simulink model "dc_ac_converter_simulation"  (R2023a)
settings: Solver=VariableStepAuto  StartTime=0.0  StopTime=sim_time  RelTol=1e-3
values from neighbouring files (symbols this model uses):
  gridfreq_rad = 2*pi*gridfreq    (= 314.159265359)    [dc_ac_converter_script.m]
  modulation = 0.8    [dc_ac_converter_script.m]
  modulation_angle = 0.123    [dc_ac_converter_script.m]
  Rd = 0.1    [dc_ac_converter_script.m]
  solver_sample_time = (1/Carrier_freq_modulation)/100    (= 6.06060606061e-06)    [dc_ac_converter_script.m]
  Vd = 3010    [dc_ac_converter_script.m]
libraries: fl_lib x22, nesl_utility x16, ee_lib x7, eeGeneralControl x6, spsTriangleGeneratorLib x1
settings Model: Creator=citcea  LastModifiedBy=citcea

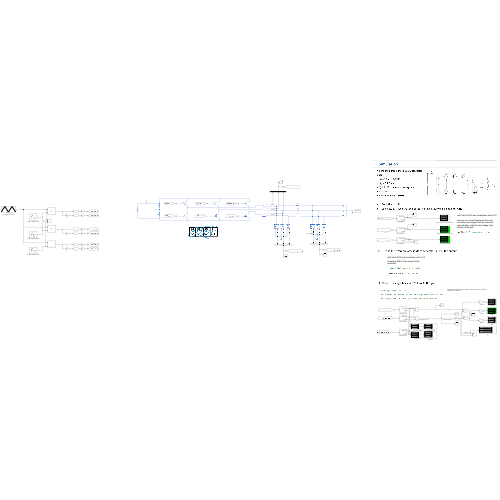
[thumbnail: Simulink's stored preview of the top-level diagram]
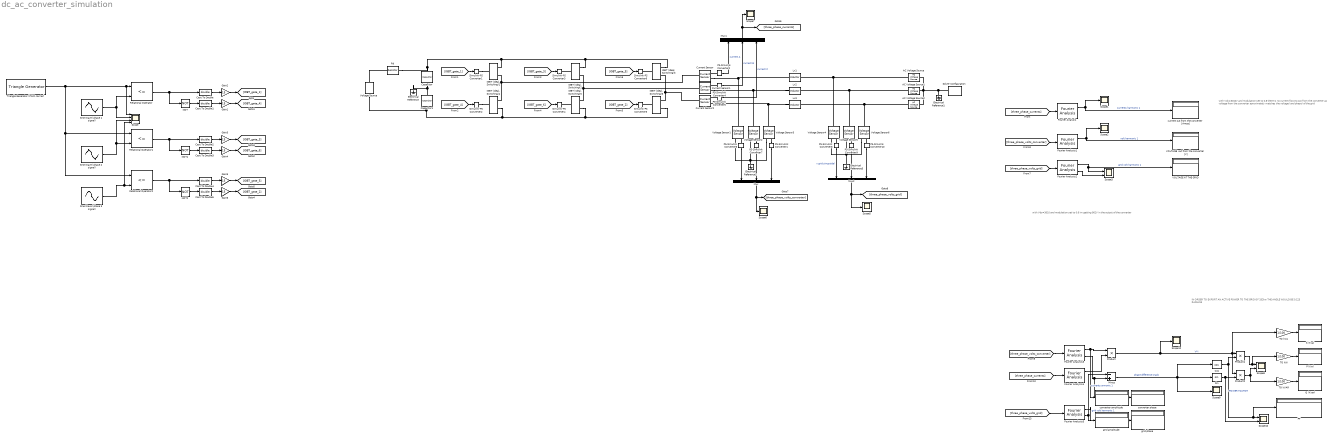
== system dc_ac_converter_simulation ==
  note: IN ORDER TO EXPORT AN ACTIVE POWER TO THE GRID OF 202kw THE ANGLE WOULD BE 0.123 RADIANS
  note: with Vdc=3010 and modulation set to 0.6
      |
      | im getting 902V in the output of the converter
  note: with Vdc=3010V and modulation set to 0.8
      |
      | there is no current flowing out from the converter as voltage from the converter aproximately matches the voltage (and phase) of the grid
  AC Voltage Source : fl_lib/Electrical/Electrical Sources/AC Voltage Source  amp=Vspeak_phase_to_ground V  shift=0 deg  frequency=gridfreq Hz  omega=0 rad/s
  AC Voltage Source1 : fl_lib/Electrical/Electrical Sources/AC Voltage Source  amp=Vspeak_phase_to_ground V  shift=120 deg  frequency=gridfreq Hz  omega=0 rad/s
  AC Voltage Source2 : fl_lib/Electrical/Electrical Sources/AC Voltage Source  amp=Vspeak_phase_to_ground V  shift=120*2 deg  frequency=gridfreq Hz  omega=0 rad/s
  Capacitor : fl_lib/Electrical/Electrical Elements/Capacitor  c=C F  r=1e-6 Ohm  g=0 1/Ohm  i_specify=off  i_priority=None  i=0 A  i_nominal_specify=off  i_nominal_unit=A  i_nominal_value=1  v_specify=off  v_priority=None  v=0 V  v_nominal_specify=off  v_nominal_unit=V  v_nominal_value=1  vc_specify=on  vc_priority=High  vc=Vd/2 V  vc_nominal_specify=off  vc_nominal_unit=V  vc_nominal_value=1
  Capacitor1 : fl_lib/Electrical/Electrical Elements/Capacitor  c=C F  r=1e-6 Ohm  g=0 1/Ohm  i_specify=off  i_priority=None  i=0 A  i_nominal_specify=off  i_nominal_unit=A  i_nominal_value=1  v_specify=off  v_priority=None  v=0 V  v_nominal_specify=off  v_nominal_unit=V  v_nominal_value=1  vc_specify=on  vc_priority=High  vc=Vd/2 V  vc_nominal_specify=off  vc_nominal_unit=V  vc_nominal_value=1
  Cast To Double{,1..5} (6 alike) : DataTypeConversion  OutDataTypeStr=double  SaturateOnIntegerOverflow=off  RndMeth=Floor
  Cos : Trigonometry  Operator=cos
  Current Sensor : fl_lib/Electrical/Electrical Sensors/Current Sensor
  Current Sensor1 : fl_lib/Electrical/Electrical Sensors/Current Sensor
  Current Sensor2 : fl_lib/Electrical/Electrical Sensors/Current Sensor
  Electrical Reference{,1..3} (4 alike) : fl_lib/Electrical/Electrical Elements/Electrical Reference
  Fourier Analysis{,1..5} (6 alike) : eeGeneralControl/Fourier Analysis  f=gridfreq  n=[1]  M0=0  Ph0=0  BufferSize=8192  Ts=solver_sample_time
      settings: LibrarySourceBlock=ee_sl_lib/General Control/Fourier Analysis
  Gain{1..6} (6 alike) : Gain  Gain=15
  IGBT (Ideal, Switching){1..6} (6 alike) : ee_lib/Semiconductors & Converters/IGBT (Ideal, Switching)  port_option=ee.enum.controlport.ps  Vf=0.8 V  Ron=0.001 Ohm  Goff=1e-5 1/Ohm  Vth=6 V  diode_param=ee.enum.converters.protectiondiode.nodynamics  diode_Vf=0.8 V  diode_Ron=0.001 Ohm  diode_Goff=1e-5 1/Ohm  diode_C=50e-9 F  diode_iRM=-235 A  diode_iF=300 A  diode_idot=-50 A/us  diode_trr_param=ee.enum.converters.diodeReverseParam.trr_factor  diode_trr_factor=3  diode_trr=15 us  diode_Qrr=1500 s*uA  ice_specify=off  ice_priority=None  ice=0 A  ice_nominal_specify=off  ice_nominal_unit=A  ice_nominal_value=1  vce_specify=off  vce_priority=None  vce=0 V  vce_nominal_specify=off  vce_nominal_unit=V  vce_nominal_value=1  vge_specify=off  vge_priority=None  vge=0 V  vge_nominal_specify=off  vge_nominal_unit=V  vge_nominal_value=1  thermal_loss_option=ee.enum.converters.thermalLossOption.constantvalues  Von_data=[0, .1, .6, .8, 1, 1.3, 1.6, 2, 2.4; 0, .1, .7, 1, 1.2, 1.5, 1.9, 2.4, 2.8] V  Tj=[298.15, 398.15] K  Iout_data=[0, .1, 1, 5, 10, 20, 40, 70, 100] A  Eon_data=[0, .0024, .024, .12, .2, .48, 1.04, 2.16, 3.24; 0, .003, .03, .15, .25, .6, 1.3, 2.7, 4.05] * 1e-3 J  Eoff_data=[0, .0007, .0066, .033, .066, .17, .33, .83, 1.5; 0, .001, .01, .05, .1, .25, .5, 1.2, 2.2] * 1e-3 J  Tj_loss=[298.15, 398.15] K  Iout_data_loss=[0, .1, 1, 5, 10, 20, 40, 70, 100] A  Eon_scalar=22.86e-3 J  Eoff_scalar=17.14e-3 J  Voff=300 V  Iout_scalar=600 A  diodeModelType=ee.enum.converters.diodeModelType.pwl  diodeTableType=ee.enum.diode.tableType.IfMat  diode_IfMat=[.07, .12, .19, 1.75, 4.24, 7.32, 11.2; .16, .3, .72, 2.14, 4.02, 6.35, 9.12] A  diode_VfMat=[.9, 1.15, 1.25, 1.5, 1.75, 2.17, 2.6, 2.85; .58, .68, .75, 1.1, 1.38, 1.77, 2.27, 2.7] V  diode_TjVec=[25, 125] degC  diode_VfVec=[.5, .7, .9, 1.3, 1.7, 2.1, 2.5] V  diode_IfVec=[.1, .2, .5, 1, 2, 4, 7, 10] A  diode_Vr=-600 V  diode_Ls=150 nH  diode_Erec=0.03 J  diode_rec_loss_model=ee.enum.diode.reverseRecoveryModel.fixed  diode_ErecVal=0 J  diode_ErecMat=zeros(2, 3) J  diode_TjrecVec=[298.15, 398.15] K  diode_IfrecVec=[.1, 1, 10] A  diode_VrecVal=10 V  diode_tFilter=1 / 1000 / 100 s  thermal_network_parameterization=ee.enum.thermalNetworkTopology.external  Rth=[.08, .5] K/W  Rth_Cauer=[.08, .1, .5] K/W  Rth_Foster=[.08, .14, .22, .16] K/W  thermal_mass_parameterization=ee.enum.thermalNetwork.timeconstant  thermal_mass=[.01, .5] J/K  thermal_mass_Cauer=[.01, .1, .5] J/K  thermal_mass_Foster=[.001, .005, .05, .5] J/K  thermal_time_constant=[.001, .2] s  thermal_time_constant_Cauer=[.001, .1, .2] s  thermal_time_constant_Foster=[7e-05, .0007, .01, .08] s  thermal_mass_initial_temperatures=[25, 25] degC  thermal_mass_initial_temperatures_Cauer=[25, 25, 25] degC  junction_thermal_mass=0.01 J/K  Tvec_initial_Foster=[25, 25, 25, 25] degC  no_thermal_network=0  junction_temperature_specify=off  junction_temperature_priority=None  junction_temperature=25 degC  junction_temperature_nominal_specify=off  junction_temperature_nominal_unit=degC  junction_temperature_nominal_value=1  Qj_specify=off  Qj_priority=None  Qj=0 W  Qj_nominal_specify=off  Qj_nominal_unit=W  Qj_nominal_value=1
  Lx1 : fl_lib/Electrical/Electrical Elements/Inductor  l=Ls H  r=RLs Ohm  g=1e-9 1/Ohm  i_specify=off  i_priority=None  i=0 A  i_nominal_specify=off  i_nominal_unit=A  i_nominal_value=1  v_specify=off  v_priority=None  v=0 V  v_nominal_specify=off  v_nominal_unit=V  v_nominal_value=1  i_L_specify=off  i_L_priority=High  i_L=0 A  i_L_nominal_specify=off  i_L_nominal_unit=A  i_L_nominal_value=1
  Lx2 : fl_lib/Electrical/Electrical Elements/Inductor  l=Ls H  r=RLs Ohm  g=1e-9 1/Ohm  i_specify=off  i_priority=None  i=0 A  i_nominal_specify=off  i_nominal_unit=A  i_nominal_value=1  v_specify=off  v_priority=None  v=0 V  v_nominal_specify=off  v_nominal_unit=V  v_nominal_value=1  i_L_specify=off  i_L_priority=High  i_L=0 A  i_L_nominal_specify=off  i_L_nominal_unit=A  i_L_nominal_value=1
  Lx3 : fl_lib/Electrical/Electrical Elements/Inductor  l=Ls H  r=RLs Ohm  g=1e-9 1/Ohm  i_specify=off  i_priority=None  i=0 A  i_nominal_specify=off  i_nominal_unit=A  i_nominal_value=1  v_specify=off  v_priority=None  v=0 V  v_nominal_specify=off  v_nominal_unit=V  v_nominal_value=1  i_L_specify=off  i_L_priority=High  i_L=0 A  i_L_nominal_specify=off  i_L_nominal_unit=A  i_L_nominal_value=1
  Minus : Sum  Inputs=-+
  Mux : Mux  Inputs=3
  Mux1 : Mux  Inputs=3
  Mux2 : Mux  Inputs=3
  NOT : Logic  Operator=NOT  IconShape=distinctive  AllPortsSameDT=off  OutDataTypeStr=boolean
  NOT1 : Logic  Operator=NOT  IconShape=distinctive  AllPortsSameDT=off  OutDataTypeStr=boolean
  NOT2 : Logic  Operator=NOT  IconShape=distinctive  AllPortsSameDT=off  OutDataTypeStr=boolean
  P (Kw) : Display
  PF : Display
  PS-Simulink Converter{1..2,4..10} (9 alike) : nesl_utility/PS-Simulink Converter  PhysicalDomain=network_engine_domain  SubClassName=ps_output  LeftPortType=input  RightPortType=output  PseudoPeriodic=off  Frequencies=[]  VectorFormat=inherit  Unit=inherit  AffineConversion=off
  Product : Product
  Product1 : Product
  Product2 : Product
  Q (Kvar) : Display
  Rd : fl_lib/Electrical/Electrical Elements/Resistor  R=Rd Ohm  i_specify=off  i_priority=None  i=0 A  i_nominal_specify=off  i_nominal_unit=A  i_nominal_value=1  v_specify=off  v_priority=None  v=0 V  v_nominal_specify=off  v_nominal_unit=V  v_nominal_value=1
  Relational Operator : RelationalOperator  Operator=<=  OutDataTypeStr=boolean  RndMeth=Simplest  InputSameDT=off
  Relational Operator1 : RelationalOperator  Operator=<=  OutDataTypeStr=boolean  RndMeth=Simplest  InputSameDT=off
  Relational Operator2 : RelationalOperator  Operator=<=  OutDataTypeStr=boolean  RndMeth=Simplest  InputSameDT=off
  S (Kva) : Display
  Scope : Scope  NumInputPorts=4
  Scope{1..2,5..7,9,12} (7 alike) : Scope
  Scope10 : Scope  NumInputPorts=2
  Scope3 : Scope  NumInputPorts=2
  Scope8 : Scope  NumInputPorts=2
  Simulink-PS Converter{1..6} (6 alike) : nesl_utility/Simulink-PS Converter  PhysicalDomain=network_engine_domain  SubClassName=ps_input  LeftPortType=input  RightPortType=output  PseudoPeriodic=off  Frequencies=[]  NoiseDistribution=none  NoiseParameters=[]  Unit=1  AffineConversion=off  FilteringAndDerivatives=provide  SimscapeFilterOrder=1  InputFilterTimeConstant=0.001  UdotUserProvided=0
  Sin : Trigonometry
  Sine Wave (phase 1 signal) : Sin  Amplitude=modulation  Frequency=gridfreq_rad  Phase=modulation_angle  SampleTime=0
  Sine Wave (phase 2 signal) : Sin  Amplitude=modulation  Frequency=gridfreq_rad  Phase=(120*pi/180)+modulation_angle  SampleTime=0
  Sine Wave (phase 3 signal) : Sin  Amplitude=modulation  Frequency=gridfreq_rad  Phase=(240*pi/180)+modulation_angle  SampleTime=0
  Solver Configuration : nesl_utility/Solver Configuration  PhysicalDomain=network_engine_domain  SubClassName=solver  LeftPortType=input  RightPortType=generic  Tones=[]  Harmonics=[]  SimulateNoise=off  Profile=off  UseLocalSampling=off  EnableSwitchedLinearOptims=on  FrequencyDomain=off  UseCCode=off  RelTol=0.001  AbsTol=0.001  MinStep=1e-09  ToWorkspace=off  RevertToSquareIcSolve=off  NumHomotopyIterations=100  PhasorMode=off  PhasorModeNumHarmonics=1  ConsistencySolver=NEWTON_XTOL_AFTER_FTOL  IndexReductionMethod=DerivativeReplacement  DoDC=off  ResidualTolerance=1e-09  ConsistencyTolSource=GLOBAL  ConsistencyAbsTol=0.001  ConsistencyRelTol=0.001  ConsistencyTolFactor=0.001  UseLocalSolver=on  LocalSolverChoice=NE_BACKWARD_EULER_ADVANCER  ResolveIndetEquations=on  FunctionEvalNumThread=1  LocalSolverSampleTime=solver_sample_time  DoFixedCost=on  MaxNonlinIter=3  MaxModeIter=2  ComputeImpulses=off  ImpulseIterations=2  LinearAlgebra=auto  LinearAlgebraNumThread=0  EquationFormulation=NE_TIME_EF  DelaysMemoryBudget=1024  AutomaticFiltering=on  FilteringTimeConstant=0.001  PartitionStorageMethod=AS_NEEDED  PartitionMemoryBudget=1024  PartitionMethod=ROBUST
  TO kVA : Gain  Gain=1/100
  TO kVAR : Gain  Gain=1/100
  TO kW : Gain  Gain=1/100
  Triangle Generator (PWM carrier) : spsTriangleGeneratorLib/Triangle Generator  Freq=Carrier_freq_modulation  Phase=0  Ts=0
  VOLTAGE  out from the converter [V] : Display
  VOLTAGE AT THE GRID : Display
  Voltage Sensor{1..6} (6 alike) : fl_lib/Electrical/Electrical Sensors/Voltage Sensor
  Voltage Source : ee_lib/Sources/Voltage Source  dc_voltage=Vd V  ac_voltage=0 V  ac_shift=0 rad  ac_frequency=60 Hz  noise_mode=ee.enum.sources.noise.Disabled  PSD=0 V^2/Hz  sample_time=1e-3 s  repeatability=ee.enum.sources.repeatability.NotRepeatable  user_seed=0  auto_seed=3890346746  i_specify=off  i_priority=None  i=0 A  i_nominal_specify=off  i_nominal_unit=A  i_nominal_value=1  v_specify=off  v_priority=None  v=0 V  v_nominal_specify=off  v_nominal_unit=V  v_nominal_value=1
  converter amplitude : Display
  converter phase : Display
  current out from the converter [Amps] : Display
  grid amplitude : Display
  grid phase : Display
  wires:
  [IGBT_gate_1] -> Simulink-PS Converter1/1
  [IGBT_gate_4] -> Simulink-PS Converter2/1
  [IGBT_gate_3] -> Simulink-PS Converter3/1
  [IGBT_gate_6] -> Simulink-PS Converter4/1
  [IGBT_gate_2] -> Simulink-PS Converter5/1
  [IGBT_gate_5] -> Simulink-PS Converter6/1
  Sine Wave (phase 1 signal)/1 -> Scope/2, Relational Operator/2
  Relational Operator/1 -> Cast To Double/1, NOT/1
  Relational Operator1/1 -> Cast To Double2/1, NOT1/1
  Sine Wave (phase 2 signal)/1 -> Scope/3, Relational Operator1/2
  Relational Operator2/1 -> Cast To Double4/1, NOT2/1
  Sine Wave (phase 3 signal)/1 -> Scope/4, Relational Operator2/2
  Triangle Generator (PWM carrier)/1 -> Relational Operator2/1, Relational Operator1/1, Scope/1, Relational Operator/1
  NOT/1 -> Cast To Double1/1
  NOT1/1 -> Cast To Double3/1
  NOT2/1 -> Cast To Double5/1
  Cast To Double/1 -> Gain2/1
  Cast To Double1/1 -> Gain1/1
  Cast To Double2/1 -> Gain3/1
  Cast To Double3/1 -> Gain4/1
  Cast To Double4/1 -> Gain5/1
  Cast To Double5/1 -> Gain6/1
  Gain2/1 -> [IGBT_gate_1]
  Gain1/1 -> [IGBT_gate_4]
  Gain3/1 -> [IGBT_gate_3]
  Gain4/1 -> [IGBT_gate_6]
  Gain5/1 -> [IGBT_gate_5]
  Gain6/1 -> [IGBT_gate_2]
  PS-Simulink Converter5/1 -> Mux1/3  "current C"
  PS-Simulink Converter6/1 -> Mux/1
  PS-Simulink Converter7/1 -> Mux/2
  PS-Simulink Converter1/1 -> Mux/3
  PS-Simulink Converter8/1 -> Mux2/1  "v grid sinusoidal"
  PS-Simulink Converter9/1 -> Mux2/2
  PS-Simulink Converter2/1 -> Mux1/1  "current A"
  Mux1/1 -> Scope7/1, [three_phase_currents]
  Mux/1 -> Scope6/1, [three_phase_volts_converter]
  PS-Simulink Converter4/1 -> Mux1/2  "current B"
  PS-Simulink Converter10/1 -> Mux2/3
  Mux2/1 -> Scope5/1, [three_phase_volts_grid]
  [three_phase_currents] -> Fourier Analysis/1
  Fourier Analysis/1 -> Scope1/1, current out from the converter [Amps]/1  "currents harmonic 1"
  [three_phase_volts_converter] -> Fourier Analysis1/1
  [three_phase_volts_grid] -> Fourier Analysis2/1
  Fourier Analysis1/1 -> Scope2/1, VOLTAGE  out from the converter [V]/1  "volt harmonic 1"
  Fourier Analysis2/1 -> Scope3/1, VOLTAGE AT THE GRID/1  "grid volt harmonic 1"
  [three_phase_volts_converter] -> Fourier Analysis3/1
  [three_phase_currents] -> Fourier Analysis4/1
  Fourier Analysis4/1 -> Product/2
  Fourier Analysis3/1 -> converter amplitude/1, Product/1  "currents armonic 1"
  Product/1 -> Scope12/1, TO kVA/1, Product2/1, Product1/1  "V*I"
  Cos/1 -> PF/1, Scope10/1, Product1/2  "POWER FACTOR"
  Sin/1 -> Scope10/2, Product2/2
  Product1/1 -> Scope8/1, TO kW/1
  Product2/1 -> Scope8/2, TO kVAR/1
  Minus/1 -> Scope9/1, Sin/1, Cos/1  "phase difference [rad]"
  Fourier Analysis2/2 -> Scope3/2
  [three_phase_volts_grid] -> Fourier Analysis5/1
  Fourier Analysis3/2 -> converter phase/1, Minus/2
  Fourier Analysis5/2 -> grid phase/1, Minus/1
  Fourier Analysis5/1 -> grid amplitude/1  "grid volt harmonic 1"
  TO kW/1 -> P (Kw)/1
  TO kVA/1 -> S (Kva)/1
  TO kVAR/1 -> Q (Kvar)/1
  connections:
  Capacitor/RConn1 -- Electrical Reference/LConn1 -- Capacitor1/LConn1
  Rd/LConn1 -- "IGBT (Ideal, Switching)3"/RConn1 -- "IGBT (Ideal, Switching)2"/RConn1 -- "IGBT (Ideal, Switching)1"/RConn1 -- Capacitor/LConn1
  Voltage Source/LConn1 -- Rd/RConn1
  Capacitor1/RConn1 -- Voltage Source/RConn1 -- "IGBT (Ideal, Switching)6"/RConn2 -- "IGBT (Ideal, Switching)5"/RConn2 -- "IGBT (Ideal, Switching)4"/RConn2
  "IGBT (Ideal, Switching)4"/RConn1 -- Current Sensor/LConn1 -- "IGBT (Ideal, Switching)1"/RConn2
  Lx2/LConn1 -- Current Sensor1/RConn2 -- Voltage Sensor2/LConn1
  "IGBT (Ideal, Switching)6"/RConn1 -- Current Sensor2/LConn1 -- "IGBT (Ideal, Switching)3"/RConn2
  AC Voltage Source/LConn1 -- Voltage Sensor4/LConn1 -- Lx1/RConn1
  AC Voltage Source1/LConn1 -- Voltage Sensor5/LConn1 -- Lx2/RConn1
  AC Voltage Source2/LConn1 -- Voltage Sensor6/LConn1 -- Lx3/RConn1
  AC Voltage Source2/RConn1 -- Solver Configuration/RConn1 -- Electrical Reference1/LConn1 -- AC Voltage Source1/RConn1 -- AC Voltage Source/RConn1
  Simulink-PS Converter2/RConn1 -- "IGBT (Ideal, Switching)4"/LConn1
  Simulink-PS Converter1/RConn1 -- "IGBT (Ideal, Switching)1"/LConn1
  "IGBT (Ideal, Switching)2"/LConn1 -- Simulink-PS Converter3/RConn1
  "IGBT (Ideal, Switching)5"/LConn1 -- Simulink-PS Converter4/RConn1
  "IGBT (Ideal, Switching)6"/LConn1 -- Simulink-PS Converter5/RConn1
  "IGBT (Ideal, Switching)3"/LConn1 -- Simulink-PS Converter6/RConn1
  Electrical Reference2/LConn1 -- Voltage Sensor3/RConn2 -- Voltage Sensor1/RConn2 -- Voltage Sensor2/RConn2
  Voltage Sensor1/LConn1 -- Lx1/LConn1 -- Current Sensor/RConn2
  "IGBT (Ideal, Switching)5"/RConn1 -- Current Sensor1/LConn1 -- "IGBT (Ideal, Switching)2"/RConn2
  Lx3/LConn1 -- Voltage Sensor3/LConn1 -- Current Sensor2/RConn2
  PS-Simulink Converter6/LConn1 -- Voltage Sensor1/RConn1
  Voltage Sensor2/RConn1 -- PS-Simulink Converter7/LConn1
  Voltage Sensor3/RConn1 -- PS-Simulink Converter1/LConn1
  PS-Simulink Converter2/LConn1 -- Current Sensor/RConn1
  PS-Simulink Converter4/LConn1 -- Current Sensor1/RConn1
  PS-Simulink Converter5/LConn1 -- Current Sensor2/RConn1
  Electrical Reference3/LConn1 -- Voltage Sensor6/RConn2 -- Voltage Sensor4/RConn2 -- Voltage Sensor5/RConn2
  PS-Simulink Converter10/LConn1 -- Voltage Sensor6/RConn1
  PS-Simulink Converter9/LConn1 -- Voltage Sensor5/RConn1
  PS-Simulink Converter8/LConn1 -- Voltage Sensor4/RConn1
